simulink library "csu_cmc_convert_measured_currents_collection_lib"  (R2014b)
settings: Solver=ode45  StartTime=0.0  StopTime=10.0  RelTol=1e-3
settings Model: Creator=escrane  LastModifiedBy=mstewart

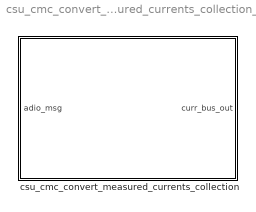
== system csu_cmc_convert_measured_currents_collection_lib ==
  csu_cmc_convert_measured_currents_collection : Subsystem
      mask Display: color('blue');text(0.05, 0.02, 'MoonEx', 'HorizontalAlignment', 'Left', 'VerticalAlignment', 'Bottom');color('red');text(0.95, 0.02, 'Autogenerated', 'HorizontalAlignment', 'Right', 'VerticalAlignment', 'Bottom');

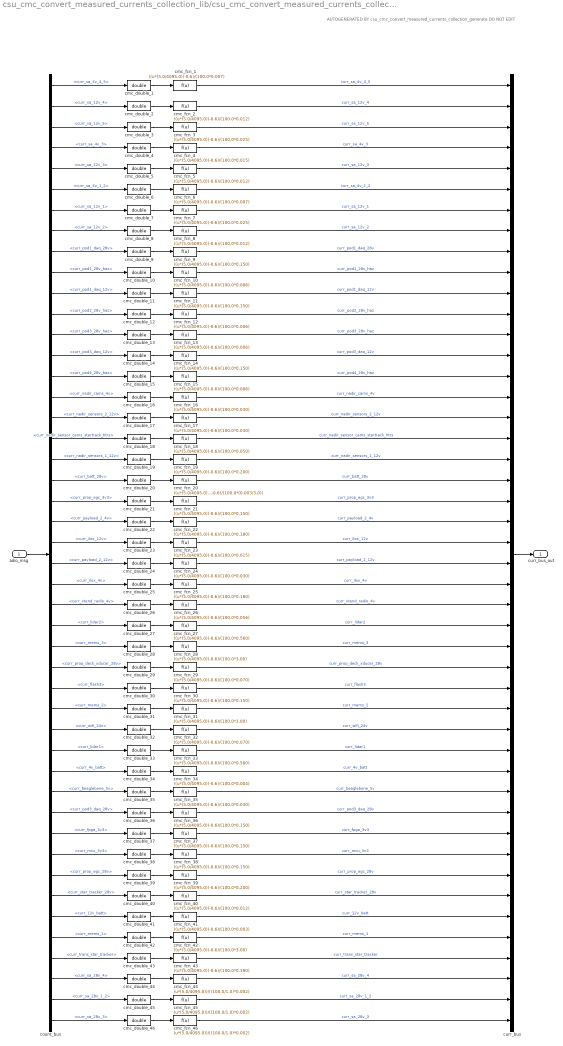
== system csu_cmc_convert_measured_currents_collection_lib/csu_cmc_convert_measured_currents_collection ==
  note: AUTOGENERATED BY csu_cmc_convert_measured_currents_collection_generate
      | DO NOT EDIT
  adio_msg : Inport
  cmc_double_{1..46} (46 alike) : DataTypeConversion  OutDataTypeStr=double
  cmc_fcn_1 : Fcn  Expr=((u*(5.0/4095.0))-0.6)/(100.0*0.007)
  cmc_fcn_{10,12..13,15} (4 alike) : Fcn  Expr=((u*(5.0/4095.0))-0.6)/(100.0*0.006)
  cmc_fcn_{9,11,14,21,30,36..38} (8 alike) : Fcn  Expr=((u*(5.0/4095.0))-0.6)/(100.0*0.150)
  cmc_fcn_{16..17,24,35} (4 alike) : Fcn  Expr=((u*(5.0/4095.0))-0.6)/(100.0*0.030)
  cmc_fcn_18 : Fcn  Expr=((u*(5.0/4095.0))-0.6)/(100.0*0.050)
  cmc_fcn_19 : Fcn  Expr=((u*(5.0/4095.0))-0.6)/(100.0*0.200)
  cmc_fcn_{2,5,8,40} (4 alike) : Fcn  Expr=((u*(5.0/4095.0))-0.6)/(100.0*0.012)
  cmc_fcn_20 : Fcn  Expr=((u*(5.0/4095.0))-0.6)/(100.0*(0.003/3.0))
  cmc_fcn_22 : Fcn  Expr=((u*(5.0/4095.0))-0.6)/(100.0*0.180)
  cmc_fcn_23 : Fcn  Expr=((u*(5.0/4095.0))-0.6)/(100.0*0.015)
  cmc_fcn_25 : Fcn  Expr=((u*(5.0/4095.0))-0.6)/(100.0*0.180)
  cmc_fcn_26 : Fcn  Expr=((u*(5.0/4095.0))-0.6)/(100.0*0.056)
  cmc_fcn_27 : Fcn  Expr=((u*(5.0/4095.0))-0.6)/(100.0*0.560)
  cmc_fcn_28 : Fcn  Expr=((u*(5.0/4095.0))-0.6)/(100.0*3.00)
  cmc_fcn_29 : Fcn  Expr=((u*(5.0/4095.0))-0.6)/(100.0*0.070)
  cmc_fcn_3 : Fcn  Expr=((u*(5.0/4095.0))-0.6)/(100.0*0.025)
  cmc_fcn_31 : Fcn  Expr=((u*(5.0/4095.0))-0.6)/(100.0*3.00)
  cmc_fcn_32 : Fcn  Expr=((u*(5.0/4095.0))-0.6)/(100.0*0.070)
  cmc_fcn_33 : Fcn  Expr=((u*(5.0/4095.0))-0.6)/(100.0*0.560)
  cmc_fcn_34 : Fcn  Expr=((u*(5.0/4095.0))-0.6)/(100.0*0.004)
  cmc_fcn_39 : Fcn  Expr=((u*(5.0/4095.0))-0.6)/(100.0*0.200)
  cmc_fcn_4 : Fcn  Expr=((u*(5.0/4095.0))-0.6)/(100.0*0.015)
  cmc_fcn_41 : Fcn  Expr=((u*(5.0/4095.0))-0.6)/(100.0*0.003)
  cmc_fcn_42 : Fcn  Expr=((u*(5.0/4095.0))-0.6)/(100.0*3.00)
  cmc_fcn_43 : Fcn  Expr=((u*(5.0/4095.0))-0.6)/(100.0*0.390)
  cmc_fcn_44 : Fcn  Expr=(u*(5.0/4095.0))/((100.0/1.0)*0.002)
  cmc_fcn_45 : Fcn  Expr=(u*(5.0/4095.0))/((100.0/1.0)*0.002)
  cmc_fcn_46 : Fcn  Expr=(u*(5.0/4095.0))/((100.0/1.0)*0.002)
  cmc_fcn_6 : Fcn  Expr=((u*(5.0/4095.0))-0.6)/(100.0*0.007)
  cmc_fcn_7 : Fcn  Expr=((u*(5.0/4095.0))-0.6)/(100.0*0.025)
  count_bus : BusSelector  OutputSignals=curr_sa_4v_4_5,curr_sa_12v_4,curr_sa_12v_5,curr_sa_4v_3,curr_sa_12v_3,curr_sa_4v_1_2,curr_sa_12v_1,curr_sa_12v_2,curr_pod1_daq_28v,curr_pod1_28v_haz,curr_pod1_daq_12v,curr_pod2_28v_haz,curr_pod3_28v_haz,curr_pod3_daq_12v,curr_pod4_28v_haz,curr_nadir_cams_4v,curr_nadir_sensors_2_12v,curr_nadir_sensor_cams_startrack_htrs,curr_nadir_sensors_1_12v,curr_batt_28v,curr_prop_egc_3v3,curr_payload_2_4v,curr_ilox_12v,curr_payload_2_12v,curr_ilox_4v,curr_xtend_radio_4v,curr_lidar2,curr_mems_3,curr_prop_deck_xducer_28v,curr_flash3,curr_mems_2,curr_wifi_24v,curr_lidar1,curr_4v_batt,curr_beaglebone_5v,curr_pod3_daq_28v,curr_fpga_3v3,curr_mcu_3v3,curr_prop_egc_28v,curr_star_tracker_28v,curr_12v_batt,curr_mems_1,curr_trans_star_tracker,curr_sa_28v_4,curr_sa_28v_1_2,curr_sa_28v_3
  curr_bus : BusCreator  Inputs=46
  curr_bus_out : Outport
  wires:
  adio_msg/1 -> count_bus/1
  curr_bus/1 -> curr_bus_out/1
  count_bus/1 -> cmc_double_1/1  "<curr_sa_4v_4_5>"
  cmc_double_1/1 -> cmc_fcn_1/1
  cmc_fcn_1/1 -> curr_bus/1  "curr_sa_4v_4_5"
  count_bus/2 -> cmc_double_2/1  "<curr_sa_12v_4>"
  cmc_double_2/1 -> cmc_fcn_2/1
  cmc_fcn_2/1 -> curr_bus/2  "curr_sa_12v_4"
  count_bus/3 -> cmc_double_3/1  "<curr_sa_12v_5>"
  cmc_double_3/1 -> cmc_fcn_3/1
  cmc_fcn_3/1 -> curr_bus/3  "curr_sa_12v_5"
  count_bus/4 -> cmc_double_4/1  "<curr_sa_4v_3>"
  cmc_double_4/1 -> cmc_fcn_4/1
  cmc_fcn_4/1 -> curr_bus/4  "curr_sa_4v_3"
  count_bus/5 -> cmc_double_5/1  "<curr_sa_12v_3>"
  cmc_double_5/1 -> cmc_fcn_5/1
  cmc_fcn_5/1 -> curr_bus/5  "curr_sa_12v_3"
  count_bus/6 -> cmc_double_6/1  "<curr_sa_4v_1_2>"
  cmc_double_6/1 -> cmc_fcn_6/1
  cmc_fcn_6/1 -> curr_bus/6  "curr_sa_4v_1_2"
  count_bus/7 -> cmc_double_7/1  "<curr_sa_12v_1>"
  cmc_double_7/1 -> cmc_fcn_7/1
  cmc_fcn_7/1 -> curr_bus/7  "curr_sa_12v_1"
  count_bus/8 -> cmc_double_8/1  "<curr_sa_12v_2>"
  cmc_double_8/1 -> cmc_fcn_8/1
  cmc_fcn_8/1 -> curr_bus/8  "curr_sa_12v_2"
  count_bus/9 -> cmc_double_9/1  "<curr_pod1_daq_28v>"
  cmc_double_9/1 -> cmc_fcn_9/1
  cmc_fcn_9/1 -> curr_bus/9  "curr_pod1_daq_28v"
  count_bus/10 -> cmc_double_10/1  "<curr_pod1_28v_haz>"
  cmc_double_10/1 -> cmc_fcn_10/1
  cmc_fcn_10/1 -> curr_bus/10  "curr_pod1_28v_haz"
  count_bus/11 -> cmc_double_11/1  "<curr_pod1_daq_12v>"
  cmc_double_11/1 -> cmc_fcn_11/1
  cmc_fcn_11/1 -> curr_bus/11  "curr_pod1_daq_12v"
  count_bus/12 -> cmc_double_12/1  "<curr_pod2_28v_haz>"
  cmc_double_12/1 -> cmc_fcn_12/1
  cmc_fcn_12/1 -> curr_bus/12  "curr_pod2_28v_haz"
  count_bus/13 -> cmc_double_13/1  "<curr_pod3_28v_haz>"
  cmc_double_13/1 -> cmc_fcn_13/1
  cmc_fcn_13/1 -> curr_bus/13  "curr_pod3_28v_haz"
  count_bus/14 -> cmc_double_14/1  "<curr_pod3_daq_12v>"
  cmc_double_14/1 -> cmc_fcn_14/1
  cmc_fcn_14/1 -> curr_bus/14  "curr_pod3_daq_12v"
  count_bus/15 -> cmc_double_15/1  "<curr_pod4_28v_haz>"
  cmc_double_15/1 -> cmc_fcn_15/1
  cmc_fcn_15/1 -> curr_bus/15  "curr_pod4_28v_haz"
  count_bus/16 -> cmc_double_16/1  "<curr_nadir_cams_4v>"
  cmc_double_16/1 -> cmc_fcn_16/1
  cmc_fcn_16/1 -> curr_bus/16  "curr_nadir_cams_4v"
  count_bus/17 -> cmc_double_17/1  "<curr_nadir_sensors_2_12v>"
  cmc_double_17/1 -> cmc_fcn_17/1
  cmc_fcn_17/1 -> curr_bus/17  "curr_nadir_sensors_2_12v"
  count_bus/18 -> cmc_double_18/1  "<curr_nadir_sensor_cams_startrack_htrs>"
  cmc_double_18/1 -> cmc_fcn_18/1
  cmc_fcn_18/1 -> curr_bus/18  "curr_nadir_sensor_cams_startrack_htrs"
  count_bus/19 -> cmc_double_19/1  "<curr_nadir_sensors_1_12v>"
  cmc_double_19/1 -> cmc_fcn_19/1
  cmc_fcn_19/1 -> curr_bus/19  "curr_nadir_sensors_1_12v"
  count_bus/20 -> cmc_double_20/1  "<curr_batt_28v>"
  cmc_double_20/1 -> cmc_fcn_20/1
  cmc_fcn_20/1 -> curr_bus/20  "curr_batt_28v"
  count_bus/21 -> cmc_double_21/1  "<curr_prop_egc_3v3>"
  cmc_double_21/1 -> cmc_fcn_21/1
  cmc_fcn_21/1 -> curr_bus/21  "curr_prop_egc_3v3"
  count_bus/22 -> cmc_double_22/1  "<curr_payload_2_4v>"
  cmc_double_22/1 -> cmc_fcn_22/1
  cmc_fcn_22/1 -> curr_bus/22  "curr_payload_2_4v"
  count_bus/23 -> cmc_double_23/1  "<curr_ilox_12v>"
  cmc_double_23/1 -> cmc_fcn_23/1
  cmc_fcn_23/1 -> curr_bus/23  "curr_ilox_12v"
  count_bus/24 -> cmc_double_24/1  "<curr_payload_2_12v>"
  cmc_double_24/1 -> cmc_fcn_24/1
  cmc_fcn_24/1 -> curr_bus/24  "curr_payload_2_12v"
  count_bus/25 -> cmc_double_25/1  "<curr_ilox_4v>"
  cmc_double_25/1 -> cmc_fcn_25/1
  cmc_fcn_25/1 -> curr_bus/25  "curr_ilox_4v"
  count_bus/26 -> cmc_double_26/1  "<curr_xtend_radio_4v>"
  cmc_double_26/1 -> cmc_fcn_26/1
  cmc_fcn_26/1 -> curr_bus/26  "curr_xtend_radio_4v"
  count_bus/27 -> cmc_double_27/1  "<curr_lidar2>"
  cmc_double_27/1 -> cmc_fcn_27/1
  cmc_fcn_27/1 -> curr_bus/27  "curr_lidar2"
  count_bus/28 -> cmc_double_28/1  "<curr_mems_3>"
  cmc_double_28/1 -> cmc_fcn_28/1
  cmc_fcn_28/1 -> curr_bus/28  "curr_mems_3"
  count_bus/29 -> cmc_double_29/1  "<curr_prop_deck_xducer_28v>"
  cmc_double_29/1 -> cmc_fcn_29/1
  cmc_fcn_29/1 -> curr_bus/29  "curr_prop_deck_xducer_28v"
  count_bus/30 -> cmc_double_30/1  "<curr_flash3>"
  cmc_double_30/1 -> cmc_fcn_30/1
  cmc_fcn_30/1 -> curr_bus/30  "curr_flash3"
  count_bus/31 -> cmc_double_31/1  "<curr_mems_2>"
  cmc_double_31/1 -> cmc_fcn_31/1
  cmc_fcn_31/1 -> curr_bus/31  "curr_mems_2"
  count_bus/32 -> cmc_double_32/1  "<curr_wifi_24v>"
  cmc_double_32/1 -> cmc_fcn_32/1
  cmc_fcn_32/1 -> curr_bus/32  "curr_wifi_24v"
  count_bus/33 -> cmc_double_33/1  "<curr_lidar1>"
  cmc_double_33/1 -> cmc_fcn_33/1
  cmc_fcn_33/1 -> curr_bus/33  "curr_lidar1"
  count_bus/34 -> cmc_double_34/1  "<curr_4v_batt>"
  cmc_double_34/1 -> cmc_fcn_34/1
  cmc_fcn_34/1 -> curr_bus/34  "curr_4v_batt"
  count_bus/35 -> cmc_double_35/1  "<curr_beaglebone_5v>"
  cmc_double_35/1 -> cmc_fcn_35/1
  cmc_fcn_35/1 -> curr_bus/35  "curr_beaglebone_5v"
  count_bus/36 -> cmc_double_36/1  "<curr_pod3_daq_28v>"
  cmc_double_36/1 -> cmc_fcn_36/1
  cmc_fcn_36/1 -> curr_bus/36  "curr_pod3_daq_28v"
  count_bus/37 -> cmc_double_37/1  "<curr_fpga_3v3>"
  cmc_double_37/1 -> cmc_fcn_37/1
  cmc_fcn_37/1 -> curr_bus/37  "curr_fpga_3v3"
  count_bus/38 -> cmc_double_38/1  "<curr_mcu_3v3>"
  cmc_double_38/1 -> cmc_fcn_38/1
  cmc_fcn_38/1 -> curr_bus/38  "curr_mcu_3v3"
  count_bus/39 -> cmc_double_39/1  "<curr_prop_egc_28v>"
  cmc_double_39/1 -> cmc_fcn_39/1
  cmc_fcn_39/1 -> curr_bus/39  "curr_prop_egc_28v"
  count_bus/40 -> cmc_double_40/1  "<curr_star_tracker_28v>"
  cmc_double_40/1 -> cmc_fcn_40/1
  cmc_fcn_40/1 -> curr_bus/40  "curr_star_tracker_28v"
  count_bus/41 -> cmc_double_41/1  "<curr_12v_batt>"
  cmc_double_41/1 -> cmc_fcn_41/1
  cmc_fcn_41/1 -> curr_bus/41  "curr_12v_batt"
  count_bus/42 -> cmc_double_42/1  "<curr_mems_1>"
  cmc_double_42/1 -> cmc_fcn_42/1
  cmc_fcn_42/1 -> curr_bus/42  "curr_mems_1"
  count_bus/43 -> cmc_double_43/1  "<curr_trans_star_tracker>"
  cmc_double_43/1 -> cmc_fcn_43/1
  cmc_fcn_43/1 -> curr_bus/43  "curr_trans_star_tracker"
  count_bus/44 -> cmc_double_44/1  "<curr_sa_28v_4>"
  cmc_double_44/1 -> cmc_fcn_44/1
  cmc_fcn_44/1 -> curr_bus/44  "curr_sa_28v_4"
  count_bus/45 -> cmc_double_45/1  "<curr_sa_28v_1_2>"
  cmc_double_45/1 -> cmc_fcn_45/1
  cmc_fcn_45/1 -> curr_bus/45  "curr_sa_28v_1_2"
  count_bus/46 -> cmc_double_46/1  "<curr_sa_28v_3>"
  cmc_double_46/1 -> cmc_fcn_46/1
  cmc_fcn_46/1 -> curr_bus/46  "curr_sa_28v_3"
